simulink model "sm_bumper_car"  (R2021b)
settings: Solver=ode45  StartTime=0.0  StopTime=10.0  MaxStep=1e-3  RelTol=1e-3  AbsTol=1e-3
model workspace: external: MATLAB File sm_bumper_car_parameters.m (data not in the file)
values from neighbouring files (symbols this model uses):
  critical_velocity = 1e-2    (= 0.01)    [sm_bumper_car_parameters.m]
  damping = 30    [sm_bumper_car_parameters.m]
  g = 9.8    [sm_bumper_car_parameters.m]
  kinetic_friction_coef = 0.2    [sm_bumper_car_parameters.m]
  static_friction_coef = 0.2    [sm_bumper_car_parameters.m]
  stiffness = 10000    [sm_bumper_car_parameters.m]
  transition_region_width = 1e-5    (= 1e-05)    [sm_bumper_car_parameters.m]
undefined symbols (not defined in the file or in its folder): BackLeft, BackRight, BackStop, Body, car, EndRamp, FrontLeft, FrontRight, Incline, LeftRail, Ramp1, Ramp2, Ramp3, Ramp4, ramp_structure, RightRail, X, Y, Z
libraries: sm_lib x131, sm_bumper_car_lib x9, nesl_utility x1
(part 1 of 2)
Description:
  | Using the Spatial Contact Force Block - Bumper Car
settings Model: Creator=The MathWorks, Inc.  LastModifiedBy=The MathWorks, Inc.
settings SolverCC: AutoScaleAbsTol=off  AlgebraicLoopSolver=TrustRegion
settings DataIOCC: ReturnWorkspaceOutputs=off
settings DebuggingCC: SymbolicDimsDataTypeCodeGenerationDiagnostic=none  SFMachineParentedDataDiag=warning
settings SimscapeCC: SimscapeLogType=all  SimscapeLogSimulationStatistics=on  SimscapeLogName=simlog_sm_bumper_car  SimscapeLogDataHistory=20000
settings ExplorerConfigSet: InternalSimMechanicsExplorerSettings="<ExplorerConfiguration><canonicalview>default</canonicalview><AnimationSetting><BasePlaybackSpeed>1.0</BasePlaybackSpeed><PlaybackSpeedFactor>1.0</PlaybackSpeedFactor></AnimationSetting><TilePanel><TileInfo><Tiles Columns=\"1\" Count=\"1\" Rows=\"1\"><Column Weight=\"1\"/><Row Weight=\"1\"/><Tile Height=\"1\" Width=\"1\" X=\"0\" Y=\"0\"/></Tiles></TileInfo><SceneInfo><SceneViewer><BGColor><R>0.800000011920928955</R><G>0.800000011920928955</G><B>0.800000011920928955</B></BGColor><Camera><DoPerspective>off</DoPerspective><Position><X>0.637508295609907183</X><Y>-0.637508296451667844</Y><Z>1.11601012334107264</Z></Position><Center><X>-0.00639254054797280813</X><Y>0.00639253970621195267</Y><Z>0.472109287183192672</Z></Center><Up><X>-0.408248290463863073</X><Y>0.408248290463863073</Y><Z>0.816496580927726145</Z></Up><ViewLimDist>1</ViewLimDist><YLim>0.759088869094848628</YLim><XLim>0.995304530142192112</XLim></Camera></SceneViewer></SceneInfo></TilePanel><MechEditorPanel><Cameras/><GfxPanelCameraMap/><VideoCreator><PlaybackSpeedRatio>1.0</PlaybackSpeedRatio><FrameRate>30</FrameRate><VideoFormat>Motion JPEG AVI</VideoFormat><FrameSize>auto</FrameSize></VideoCreator></MechEditorPanel></ExplorerConfiguration>"

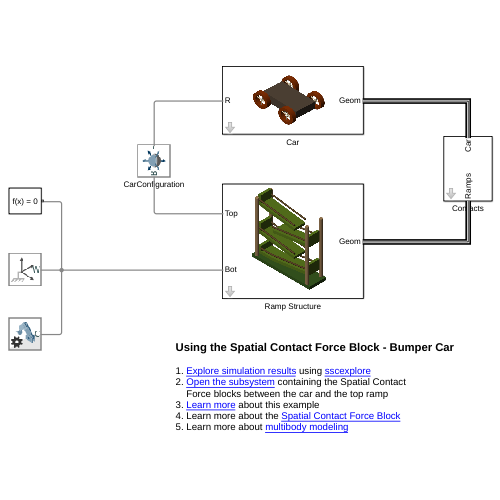
[thumbnail: Simulink's stored preview of the top-level diagram]
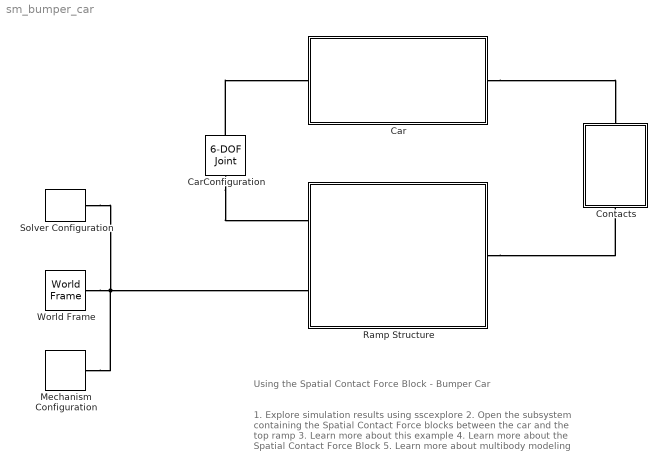
== system sm_bumper_car ==
  note: Using the Spatial Contact Force Block - Bumper Car
  note: 1. Explore simulation results using sscexplore
      | 2. Open the subsystem containing the Spatial Contact
      | Force blocks between the car and the top ramp
      | 3. Learn more about this example
      | 4. Learn more about the Spatial Contact Force Block
      | 5. Learn more about multibody modeling
  Car : Subsystem  mask{l=car.body.length, w=car.body.width, h=car.body.height, m=car.body.mass, body_color=car.body.color, wheel_radius=car.wheel.radius, wheel_width=car.wheel.thickness, wheel_m=car.wheel.mass, wheel_color=car.wheel.color, wheel_spoke_color=car.wheel.spoke.color}
      mask prompts: l "Length (cm)"; w "Width (cm)"; h "Height (cm)"; m "Body Mass (kg)"; body_color "Car Body Color"; wheel_radius "Radius"; wheel_width "Thickness"; wheel_m "Wheel Mass (kg)"; wheel_color "Wheel Color"; wheel_spoke_color "Wheel Spoke Color"
      mask init:
      | axle_len               = .85 * l;
      | axle_radius            = axle_len / 30;
      | wheel_inner_radius     = .67 * wheel_radius;
      | wheel_spoke_thickness = axle_radius / 2;
      | 
      | front_wheel_pos  = l * .12;
      | back_wheel_pos   = l * .88;
      | wheel_separation = axle_len;
      mask DialogControl BodyGroupVar Prompt: Body
      mask DialogControl BodyDimGroupVar Prompt: Dimensions
      mask DialogControl BodyInertiaGroupVar Prompt: Inertia
      mask DialogControl BodyGraphicGroupVar Prompt: Graphic
      mask DialogControl WheelGroupVar Prompt: Wheels
      mask DialogControl WheelDimGroupVar Prompt: Dimensions
      mask DialogControl WheelInertiaGroupVar Prompt: Inertia
      mask DialogControl WheelGraphicGroupVar Prompt: Graphic
      mask Display: image(fullfile(matlabroot,'toolbox','physmod','sm','smdemos','bumper_car','images','sm_bumper_car_car.png'));
  CarConfiguration : sm_lib/Joints/6-DOF Joint  JointMode=Normal  SenseConstraintForce=off  SenseConstraintForceX=off  SenseConstraintForceY=off  SenseConstraintForceZ=off  SenseConstraintTorque=off  SenseConstraintTorqueX=off  SenseConstraintTorqueY=off  SenseConstraintTorqueZ=off  SenseTotalForce=off  SenseTotalForceX=off  SenseTotalForceY=off  SenseTotalForceZ=off  SenseTotalTorque=off  SenseTotalTorqueX=off  SenseTotalTorqueY=off  SenseTotalTorqueZ=off  CompositeWrenchDir=FollowerOnBase  CompositeWrenchFrame=BaseFrame  PxEquilibriumPosition=0  PxEquilibriumPositionUnits=m  PxSpringStiffness=0  PxSpringStiffnessUnits=N/m  PxDampingCoefficient=0  PxDampingCoefficientUnits=N/(m/s)  PxTorqueActuationMode=NoTorque  PxMotionActuationMode=ComputedMotion  PxSensePosition=off  PxSenseVelocity=off  PxSenseAcceleration=off  PxSenseTorqueForce=off  PxSenseLowerLimitTorqueForce=off  PxSenseUpperLimitTorqueForce=off  PxLowerLimitSpecify=off  PxLowerLimitBound=-1  PxLowerLimitBoundUnits=m  PxLowerLimitStiffness=1e6  PxLowerLimitStiffnessUnits=N/m  PxLowerLimitDamping=1e3  PxLowerLimitDampingUnits=N/(m/s)  PxLowerLimitTransitionRegionWidth=1e-4  PxLowerLimitTransitionRegionWidthUnits=m  PxUpperLimitSpecify=off  PxUpperLimitBound=1  PxUpperLimitBoundUnits=m  PxUpperLimitStiffness=1e6  PxUpperLimitStiffnessUnits=N/m  PxUpperLimitDamping=1e3  PxUpperLimitDampingUnits=N/(m/s)  PxUpperLimitTransitionRegionWidth=1e-4  PxUpperLimitTransitionRegionWidthUnits=m  PxPositionTargetSpecify=on  PxPositionTargetPriority=High  PxPositionTargetValue=car.start_dist  PxPositionTargetValueUnits=cm  PxVelocityTargetSpecify=off  PxVelocityTargetPriority=High  PxVelocityTargetValue=0  PxVelocityTargetValueUnits=m/s  PyEquilibriumPosition=0  PyEquilibriumPositionUnits=m  PySpringStiffness=0  PySpringStiffnessUnits=N/m  PyDampingCoefficient=0  PyDampingCoefficientUnits=N/(m/s)  PyTorqueActuationMode=NoTorque  PyMotionActuationMode=ComputedMotion  PySensePosition=off  PySenseVelocity=off  PySenseAcceleration=off  PySenseTorqueForce=off  PySenseLowerLimitTorqueForce=off  PySenseUpperLimitTorqueForce=off  PyLowerLimitSpecify=off  PyLowerLimitBound=-1  PyLowerLimitBoundUnits=m  PyLowerLimitStiffness=1e6  PyLowerLimitStiffnessUnits=N/m  PyLowerLimitDamping=1e3  PyLowerLimitDampingUnits=N/(m/s)  PyLowerLimitTransitionRegionWidth=1e-4  PyLowerLimitTransitionRegionWidthUnits=m  PyUpperLimitSpecify=off  PyUpperLimitBound=1  PyUpperLimitBoundUnits=m  PyUpperLimitStiffness=1e6  PyUpperLimitStiffnessUnits=N/m  PyUpperLimitDamping=1e3  PyUpperLimitDampingUnits=N/(m/s)  PyUpperLimitTransitionRegionWidth=1e-4  PyUpperLimitTransitionRegionWidthUnits=m  PyPositionTargetSpecify=off  PyPositionTargetPriority=High  PyPositionTargetValue=0  PyPositionTargetValueUnits=m  PyVelocityTargetSpecify=off  PyVelocityTargetPriority=High  PyVelocityTargetValue=0  PyVelocityTargetValueUnits=m/s  PzEquilibriumPosition=0  PzEquilibriumPositionUnits=m  PzSpringStiffness=0  PzSpringStiffnessUnits=N/m  PzDampingCoefficient=0  PzDampingCoefficientUnits=N/(m/s)  PzTorqueActuationMode=NoTorque  PzMotionActuationMode=ComputedMotion  PzSensePosition=off  PzSenseVelocity=off  PzSenseAcceleration=off  PzSenseTorqueForce=off  PzSenseLowerLimitTorqueForce=off  PzSenseUpperLimitTorqueForce=off  PzLowerLimitSpecify=off  PzLowerLimitBound=-1  PzLowerLimitBoundUnits=m  PzLowerLimitStiffness=1e6  PzLowerLimitStiffnessUnits=N/m  PzLowerLimitDamping=1e3  PzLowerLimitDampingUnits=N/(m/s)  PzLowerLimitTransitionRegionWidth=1e-4  PzLowerLimitTransitionRegionWidthUnits=m  PzUpperLimitSpecify=off  PzUpperLimitBound=1  PzUpperLimitBoundUnits=m  PzUpperLimitStiffness=1e6  PzUpperLimitStiffnessUnits=N/m  PzUpperLimitDamping=1e3  PzUpperLimitDampingUnits=N/(m/s)  PzUpperLimitTransitionRegionWidth=1e-4  PzUpperLimitTransitionRegionWidthUnits=m  PzPositionTargetSpecify=on  PzPositionTargetPriority=High  PzPositionTargetValue=car.start_height  PzPositionTargetValueUnits=cm  PzVelocityTargetSpecify=off  PzVelocityTargetPriority=High  PzVelocityTargetValue=0  PzVelocityTargetValueUnits=m/s  SphDefPosRotationMethod=None  SphDefPosRotationAngleUnits=deg  SphDefPosRotationStandardAxis=+Z  SphDefPosRotationAngle=0.0  SphDefPosRotationArbitraryAxis=[0 0 1]  SphDefPosFollAlignAxisA=+X  SphDefPosBaseAlignAxisA=+Y  SphDefPosFollAlignAxisB=+Y  SphDefPosBaseAlignAxisB=+Z  SphDefPosRotationSequenceAxes=FollowerAxes  SphDefPosRotationSequence=XYX  SphDefPosRotationSequenceAngles=[0 0 0]  SphDefPosRotationSequenceAnglesUnits=deg  SphDefPosRotationMatrix=[1 0 0; 0 1 0; 0 0 1]  SphEqPosRotationMethod=None  SphEqPosRotationAngleUnits=deg  SphEqPosRotationStandardAxis=+Z  SphEqPosRotationAngle=0.0  SphEqPosRotationArbitraryAxis=[0 0 1]  SphEqPosFollAlignAxisA=+X  SphEqPosBaseAlignAxisA=+Y  SphEqPosFollAlignAxisB=+Y  SphEqPosBaseAlignAxisB=+Z  SphEqPosRotationSequenceAxes=FollowerAxes  SphEqPosRotationSequence=XYX  SphEqPosRotationSequenceAngles=[0 0 0]  SphEqPosRotationSequenceAnglesUnits=deg  SphEqPosRotationMatrix=[1 0 0; 0 1 0; 0 0 1]  SphSpringStiffness=0  SphSpringStiffnessUnits=N*m/deg  SphDampingCoefficient=0  SphDampingCoefficientUnits=N*m/(deg/s)  SphActuateTorqueX=off  SphActuateTorqueY=off  SphActuateTorqueZ=off  SphActuateTorque=off  SphTorqueActuationMode=NoTorque  SphMotionActuationMode=ComputedMotion  SphActuationFrame=BaseFrame  SphSensePosition=off  SphSenseVelocityX=off  SphSenseVelocityY=off  SphSenseVelocityZ=off  SphSenseVelocity=off  SphSenseAccelerationX=off  SphSenseAccelerationY=off  SphSenseAccelerationZ=off  SphSenseAcceleration=off  SphSenseTorqueX=off  SphSenseTorqueY=off  SphSenseTorqueZ=off  SphSenseTorqueForce=off  SphSenseLowerLimitTorqueMag=off  SphSenseUpperLimitTorqueMag=off  SphSensingFrame=BaseFrame  SphLowerLimitSpecify=off  SphLowerLimitBound=15  SphLowerLimitBoundUnits=deg  SphLowerLimitStiffness=1e4  SphLowerLimitStiffnessUnits=N*m/deg  SphLowerLimitDamping=10  SphLowerLimitDampingUnits=N*m/(deg/s)  SphLowerLimitTransitionRegionWidth=0.1  SphLowerLimitTransitionRegionWidthUnits=deg  SphUpperLimitSpecify=off  SphUpperLimitBound=45  SphUpperLimitBoundUnits=deg  SphUpperLimitStiffness=1e4  SphUpperLimitStiffnessUnits=N*m/deg  SphUpperLimitDamping=10  SphUpperLimitDampingUnits=N*m/(deg/s)  SphUpperLimitTransitionRegionWidth=0.1  SphUpperLimitTransitionRegionWidthUnits=deg  SphPositionTargetRotationMethod=StandardAxis  SphPositionTargetRotationAngleUnits=deg  SphPositionTargetRotationStandardAxis=-Y  SphPositionTargetRotationAngle=car.start_pitch  SphPositionTargetRotationArbitraryAxis=[0 0 1]  SphPositionTargetFollAlignAxisA=+X  SphPositionTargetBaseAlignAxisA=+Y  SphPositionTargetFollAlignAxisB=+Y  SphPositionTargetBaseAlignAxisB=+Z  SphPositionTargetRotationSequenceAxes=FollowerAxes  SphPositionTargetRotationSequence=XYX  SphPositionTargetRotationSequenceAngles=[0 0 0]  SphPositionTargetRotationSequenceAnglesUnits=deg  SphPositionTargetRotationMatrix=[1 0 0; 0 1 0; 0 0 1]  SphPositionTargetSpecify=on  SphPositionTargetPriority=High  SphVelocityTargetValue=[0 0 0]  SphVelocityTargetValueUnits=deg/s  SphVelocityTargetSpecify=off  SphVelocityTargetPriority=High  SphVelocityTargetInFollowerFrame=on
  Contacts : Subsystem  mask{k=stiffness, b=damping, tau=transition_region_width, mus=static_friction_coef, muk=kinetic_friction_coef, cv=critical_velocity}
      mask prompts: k "Stiffness (N/m)"; b "Damping (N/(m/s))"; tau "Transition Region Width (m)"; mus "Coefficient of Static Friction"; muk "Coefficient of Kinetic Friction"; cv "Critical Velocity (m/s)"
  Mechanism Configuration : sm_lib/Utilities/Mechanism Configuration  UniformGravity=Constant  GravityVector=[0 0 -g]  GravityUnits=m/s^2  LinearizationDelta=0.001  JointModeTransitionNonlinearIterations=2
  Ramp Structure : Subsystem  mask{w=ramp_structure.width, l=ramp_structure.length, ramp_angle=ramp_structure.ramp.angle, surface_color=ramp_structure.ramp.color, rail_color=ramp_structure.rail.color, pillar_color=ramp_structure.pillar.color, base_color=ramp_structure.base.color}
      mask prompts: w "Width (cm)"; l "Length (cm)"; ramp_angle "Ramp Angle (deg)"; surface_color "Surface Color"; rail_color "Rail Color"; pillar_color "Pillar Color"; base_color "Base Color"
      mask init:
      | ramp.angle = ramp_angle;
      | theta_ = deg2rad(ramp.angle);
      | 
      | ramp.w       = w;
      | ramp.h       = ramp.w / 4;
      | 
      | wall.h        = ramp.w;
      | 
      | dropoff_h     = .75 * ramp.w;
      | dropoff_dist  = 1.5 * ramp.w;
      | 
      | ramp.l        = (l - dropoff_dist - sin(theta_)*ramp.h/2)...
      |                 / cos(theta_);
      | 
      | rail.r        = .28 * ramp.h;
      | rail.l        = ramp.l;
      | 
      | rail.h = 1.5 * ramp.h;
      | 
      | end_ramp.l = dropoff_dist + ramp.h;
      | 
      | ramp.w = ramp.w + 2 * rail.r;
      mask DialogControl ParameterGroupVar Prompt: Geometry
      mask DialogControl GraphicsGroupVar Prompt: Graphic
      mask Display: image(fullfile(matlabroot,'toolbox','physmod','sm','smdemos','bumper_car','images','sm_bumper_car_ramp_structure.png'));
  Solver Configuration : nesl_utility/Solver Configuration  PhysicalDomain=network_engine_domain  SubClassName=solver  LeftPortType=input  RightPortType=generic  Tones=[]  Harmonics=[]  SimulateNoise=off  Profile=off  UseLocalSampling=off  EnableSwitchedLinearOptims=on  FrequencyDomain=off  UseCCode=off  RelTol=0.001  AbsTol=1e-06  MinStep=1e-09  ToWorkspace=off  RevertToSquareIcSolve=off  NumHomotopyIterations=100  PhasorMode=off  PhasorModeNumHarmonics=1  DoDC=off  ResidualTolerance=1e-09  UseLocalSolver=off  LocalSolverChoice=NE_BACKWARD_EULER_ADVANCER  LocalSolverSampleTime=0.001  DoFixedCost=off  MaxNonlinIter=3  MaxModeIter=2  ComputeImpulses=off  ImpulseIterations=2  LinearAlgebra=Sparse  EquationFormulation=NE_TIME_EF  DelaysMemoryBudget=1024  AutomaticFiltering=on  FilteringTimeConstant=0.001  PartitionStorageMethod=AS_NEEDED  PartitionMemoryBudget=1024  PartitionMethod=FAST
      settings: SourceProductBaseCode=PW,SS
  World Frame : sm_lib/Frames and Transforms/World Frame
  connections:
  Solver Configuration/RConn1 -- Ramp Structure/LConn2 -- Mechanism Configuration/RConn1 -- World Frame/RConn1
  CarConfiguration/RConn1 -- Car/LConn1
  CarConfiguration/LConn1 -- Ramp Structure/LConn1
  Ramp Structure/RConn1 -- Contacts/LConn1
  Car/RConn1 -- Contacts/RConn1

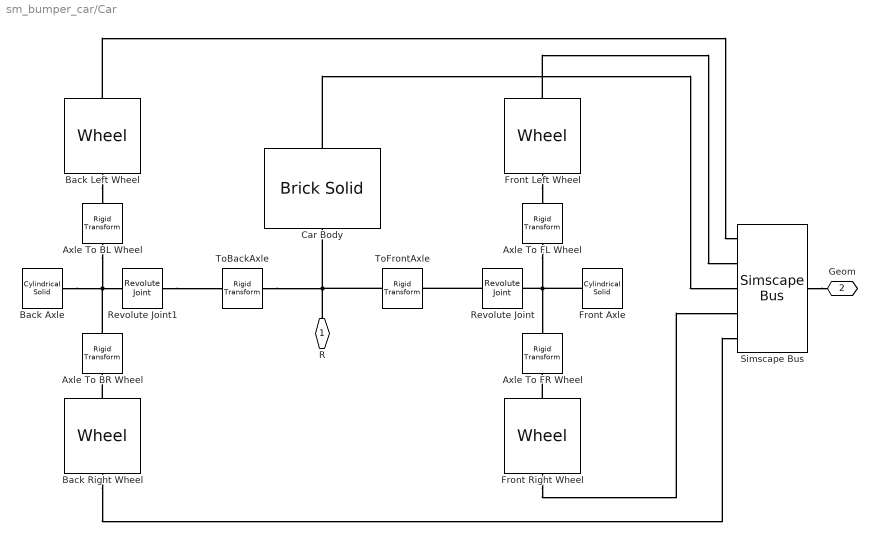
== system sm_bumper_car/Car ==
  Axle To BL Wheel : sm_lib/Frames and Transforms/Rigid Transform  TranslationMethod=StandardAxis  TranslationStandardOffset=wheel_separation/2  TranslationLengthUnit=cm  TranslationStandardAxis=-Z  TranslationCartesianOffset=[0 0 0]  TranslationROffset=0  TranslationROffsetUnits=m  TranslationZOffset=0  TranslationZOffsetUnits=m  TranslationThetaOffset=0  TranslationThetaOffsetUnits=deg  RotationMethod=None  RotationAngleUnits=deg  RotationStandardAxis=+Z  RotationAngle=0.0  RotationArbitraryAxis=[0 0 1]  FollAlignAxisA=+X  BaseAlignAxisA=+Y  FollAlignAxisB=+Y  BaseAlignAxisB=+Z  RotationSequenceAxes=FollowerAxes  RotationSequence=XYX  RotationSequenceAngles=[0 0 0]  RotationSequenceAnglesUnits=deg  RotationMatrix=[1 0 0; 0 1 0; 0 0 1]
  Axle To BR Wheel : sm_lib/Frames and Transforms/Rigid Transform  TranslationMethod=StandardAxis  TranslationStandardOffset=wheel_separation/2  TranslationLengthUnit=cm  TranslationStandardAxis=+Z  TranslationCartesianOffset=[0 0 0]  TranslationROffset=0  TranslationROffsetUnits=m  TranslationZOffset=0  TranslationZOffsetUnits=m  TranslationThetaOffset=0  TranslationThetaOffsetUnits=deg  RotationMethod=None  RotationAngleUnits=deg  RotationStandardAxis=+Z  RotationAngle=0.0  RotationArbitraryAxis=[0 0 1]  FollAlignAxisA=+X  BaseAlignAxisA=+Y  FollAlignAxisB=+Y  BaseAlignAxisB=+Z  RotationSequenceAxes=FollowerAxes  RotationSequence=XYX  RotationSequenceAngles=[0 0 0]  RotationSequenceAnglesUnits=deg  RotationMatrix=[1 0 0; 0 1 0; 0 0 1]
  Axle To FL Wheel : sm_lib/Frames and Transforms/Rigid Transform  TranslationMethod=StandardAxis  TranslationStandardOffset=wheel_separation/2  TranslationLengthUnit=cm  TranslationStandardAxis=-Z  TranslationCartesianOffset=[0 0 0]  TranslationROffset=0  TranslationROffsetUnits=m  TranslationZOffset=0  TranslationZOffsetUnits=m  TranslationThetaOffset=0  TranslationThetaOffsetUnits=deg  RotationMethod=None  RotationAngleUnits=deg  RotationStandardAxis=+Z  RotationAngle=0.0  RotationArbitraryAxis=[0 0 1]  FollAlignAxisA=+X  BaseAlignAxisA=+Y  FollAlignAxisB=+Y  BaseAlignAxisB=+Z  RotationSequenceAxes=FollowerAxes  RotationSequence=XYX  RotationSequenceAngles=[0 0 0]  RotationSequenceAnglesUnits=deg  RotationMatrix=[1 0 0; 0 1 0; 0 0 1]
  Axle To FR Wheel : sm_lib/Frames and Transforms/Rigid Transform  TranslationMethod=StandardAxis  TranslationStandardOffset=wheel_separation/2  TranslationLengthUnit=cm  TranslationStandardAxis=+Z  TranslationCartesianOffset=[0 0 0]  TranslationROffset=0  TranslationROffsetUnits=m  TranslationZOffset=0  TranslationZOffsetUnits=m  TranslationThetaOffset=0  TranslationThetaOffsetUnits=deg  RotationMethod=None  RotationAngleUnits=deg  RotationStandardAxis=+Z  RotationAngle=0.0  RotationArbitraryAxis=[0 0 1]  FollAlignAxisA=+X  BaseAlignAxisA=+Y  FollAlignAxisB=+Y  BaseAlignAxisB=+Z  RotationSequenceAxes=FollowerAxes  RotationSequence=XYX  RotationSequenceAngles=[0 0 0]  RotationSequenceAnglesUnits=deg  RotationMatrix=[1 0 0; 0 1 0; 0 0 1]
  Back Axle : sm_lib/Body Elements/Cylindrical Solid  GraphicAmbientColor=[0.15 0.15 0.15 1.0]  BasedOnType=Density  CenterOfMass=[0 0 0]  CenterOfMassUnits=m  GraphicDiffuseColor=wheel_spoke_color  CylinderLength=axle_len  CylinderLengthUnits=cm  CylinderRadius=axle_radius  CylinderRadiusUnits=cm  Density=0  DensityUnits=kg/m^3  DoExposeReferenceFrame=on  GraphicEmissiveColor=[0.0 0.0 0.0 1.0]  ExportEntireGeometry=off  SerializedFrames=<Frames/>  MarkerShape=Sphere  MarkerSize=10  GraphicType=FromGeometry  InertiaType=CalculateFromGeometry  Mass=1  MassUnits=kg  MomentsOfInertia=[1 1 1]  MomentsOfInertiaUnits=kg*m^2  GraphicOpacity=1.0  ProductsOfInertia=[0 0 0]  ProductsOfInertiaUnits=kg*m^2  GraphicShininess=75  GraphicSpecularColor=[0.5 0.5 0.5 1.0]  GraphicVisPropType=SimpleVisualProperties
  Back Left Wheel : sm_bumper_car_lib/Wheel  r=wheel_radius  rin=wheel_inner_radius  spoke_r=wheel_spoke_thickness  W=wheel_width  m=wheel_m  color=wheel_color  spoke_color=wheel_spoke_color
      settings: SourceProductBaseCode=MS
  Back Right Wheel : sm_bumper_car_lib/Wheel  r=wheel_radius  rin=wheel_inner_radius  spoke_r=wheel_spoke_thickness  W=wheel_width  m=wheel_m  color=wheel_color  spoke_color=wheel_spoke_color
      settings: SourceProductBaseCode=MS
  Car Body : sm_lib/Body Elements/Brick Solid  GraphicAmbientColor=[0.15 0.15 0.15 1.0]  BasedOnType=Mass  BrickDimensions=[l w h]  BrickDimensionUnits=cm  CenterOfMass=[0 0 0]  CenterOfMassUnits=cm  GraphicDiffuseColor=body_color  Density=1000  DensityUnits=kg/m^3  DoExposeReferenceFrame=on  GraphicEmissiveColor=[0.0 0.0 0.0 1.0]  ExportEntireGeometry=on  SerializedFrames=<Frames/>  MarkerShape=Sphere  MarkerSize=10  GraphicType=FromGeometry  InertiaType=CalculateFromGeometry  Mass=m  MassUnits=kg  MomentsOfInertia=[1 1 1]  MomentsOfInertiaUnits=kg*m^2  GraphicOpacity=1.0  ProductsOfInertia=[0 0 0]  ProductsOfInertiaUnits=kg*m^2  GraphicShininess=75  GraphicSpecularColor=[0.5 0.5 0.5 1.0]  GraphicVisPropType=SimpleVisualProperties
  Front Axle : sm_lib/Body Elements/Cylindrical Solid  GraphicAmbientColor=[0.15 0.15 0.15 1.0]  BasedOnType=Density  CenterOfMass=[0 0 0]  CenterOfMassUnits=m  GraphicDiffuseColor=wheel_spoke_color  CylinderLength=axle_len  CylinderLengthUnits=cm  CylinderRadius=axle_radius  CylinderRadiusUnits=cm  Density=0  DensityUnits=kg/m^3  DoExposeReferenceFrame=on  GraphicEmissiveColor=[0.0 0.0 0.0 1.0]  ExportEntireGeometry=off  SerializedFrames=<Frames/>  MarkerShape=Sphere  MarkerSize=10  GraphicType=FromGeometry  InertiaType=CalculateFromGeometry  Mass=1  MassUnits=kg  MomentsOfInertia=[1 1 1]  MomentsOfInertiaUnits=kg*m^2  GraphicOpacity=1.0  ProductsOfInertia=[0 0 0]  ProductsOfInertiaUnits=kg*m^2  GraphicShininess=75  GraphicSpecularColor=[0.5 0.5 0.5 1.0]  GraphicVisPropType=SimpleVisualProperties
  Front Left Wheel : sm_bumper_car_lib/Wheel  r=wheel_radius  rin=wheel_inner_radius  spoke_r=wheel_spoke_thickness  W=wheel_width  m=wheel_m  color=wheel_color  spoke_color=wheel_spoke_color
      settings: SourceProductBaseCode=MS
  Front Right Wheel : sm_bumper_car_lib/Wheel  r=wheel_radius  rin=wheel_inner_radius  spoke_r=wheel_spoke_thickness  W=wheel_width  m=wheel_m  color=wheel_color  spoke_color=wheel_spoke_color
      settings: SourceProductBaseCode=MS
  Revolute Joint : sm_lib/Joints/Revolute Joint  JointMode=Normal  SenseConstraintForce=off  SenseConstraintForceX=off  SenseConstraintForceY=off  SenseConstraintForceZ=off  SenseConstraintTorque=off  SenseConstraintTorqueX=off  SenseConstraintTorqueY=off  SenseConstraintTorqueZ=off  SenseTotalForce=off  SenseTotalForceX=off  SenseTotalForceY=off  SenseTotalForceZ=off  SenseTotalTorque=off  SenseTotalTorqueX=off  SenseTotalTorqueY=off  SenseTotalTorqueZ=off  CompositeWrenchDir=FollowerOnBase  CompositeWrenchFrame=BaseFrame  EquilibriumPosition=0  EquilibriumPositionUnits=deg  SpringStiffness=0  SpringStiffnessUnits=N*m/deg  DampingCoefficient=0  DampingCoefficientUnits=N*m/(deg/s)  TorqueActuationMode=NoTorque  MotionActuationMode=ComputedMotion  SensePosition=off  SenseVelocity=off  SenseAcceleration=off  SenseTorqueForce=off  SenseLowerLimitTorqueForce=off  SenseUpperLimitTorqueForce=off  LowerLimitSpecify=off  LowerLimitBound=-90  LowerLimitBoundUnits=deg  LowerLimitStiffness=1e4  LowerLimitStiffnessUnits=N*m/deg  LowerLimitDamping=10  LowerLimitDampingUnits=N*m/(deg/s)  LowerLimitTransitionRegionWidth=0.1  LowerLimitTransitionRegionWidthUnits=deg  UpperLimitSpecify=off  UpperLimitBound=90  UpperLimitBoundUnits=deg  UpperLimitStiffness=1e4  UpperLimitStiffnessUnits=N*m/deg  UpperLimitDamping=10  UpperLimitDampingUnits=N*m/(deg/s)  UpperLimitTransitionRegionWidth=0.1  UpperLimitTransitionRegionWidthUnits=deg  PositionTargetSpecify=off  PositionTargetPriority=High  PositionTargetValue=0  PositionTargetValueUnits=deg  VelocityTargetSpecify=off  VelocityTargetPriority=High  VelocityTargetValue=0  VelocityTargetValueUnits=deg/s
  Revolute Joint1 : sm_lib/Joints/Revolute Joint  JointMode=Normal  SenseConstraintForce=off  SenseConstraintForceX=off  SenseConstraintForceY=off  SenseConstraintForceZ=off  SenseConstraintTorque=off  SenseConstraintTorqueX=off  SenseConstraintTorqueY=off  SenseConstraintTorqueZ=off  SenseTotalForce=off  SenseTotalForceX=off  SenseTotalForceY=off  SenseTotalForceZ=off  SenseTotalTorque=off  SenseTotalTorqueX=off  SenseTotalTorqueY=off  SenseTotalTorqueZ=off  CompositeWrenchDir=FollowerOnBase  CompositeWrenchFrame=BaseFrame  EquilibriumPosition=0  EquilibriumPositionUnits=deg  SpringStiffness=0  SpringStiffnessUnits=N*m/deg  DampingCoefficient=0  DampingCoefficientUnits=N*m/(deg/s)  TorqueActuationMode=NoTorque  MotionActuationMode=ComputedMotion  SensePosition=off  SenseVelocity=off  SenseAcceleration=off  SenseTorqueForce=off  SenseLowerLimitTorqueForce=off  SenseUpperLimitTorqueForce=off  LowerLimitSpecify=off  LowerLimitBound=-90  LowerLimitBoundUnits=deg  LowerLimitStiffness=1e4  LowerLimitStiffnessUnits=N*m/deg  LowerLimitDamping=10  LowerLimitDampingUnits=N*m/(deg/s)  LowerLimitTransitionRegionWidth=0.1  LowerLimitTransitionRegionWidthUnits=deg  UpperLimitSpecify=off  UpperLimitBound=90  UpperLimitBoundUnits=deg  UpperLimitStiffness=1e4  UpperLimitStiffnessUnits=N*m/deg  UpperLimitDamping=10  UpperLimitDampingUnits=N*m/(deg/s)  UpperLimitTransitionRegionWidth=0.1  UpperLimitTransitionRegionWidthUnits=deg  PositionTargetSpecify=off  PositionTargetPriority=High  PositionTargetValue=0  PositionTargetValueUnits=deg  VelocityTargetSpecify=off  VelocityTargetPriority=High  VelocityTargetValue=0  VelocityTargetValueUnits=deg/s
  Simscape Bus : SimscapeBus  HierarchyStrings=BackLeft;FrontLeft;Body;FrontRight;BackRight
  ToBackAxle : sm_lib/Frames and Transforms/Rigid Transform  TranslationMethod=StandardAxis  TranslationStandardOffset=l/2 - back_wheel_pos  TranslationLengthUnit=cm  TranslationStandardAxis=+X  TranslationCartesianOffset=[0 0 0]  TranslationROffset=0  TranslationROffsetUnits=m  TranslationZOffset=0  TranslationZOffsetUnits=m  TranslationThetaOffset=0  TranslationThetaOffsetUnits=deg  RotationMethod=AlignedAxes  RotationAngleUnits=deg  RotationStandardAxis=+Z  RotationAngle=0.0  RotationArbitraryAxis=[0 0 1]  FollAlignAxisA=+Y  BaseAlignAxisA=+Z  FollAlignAxisB=+Z  BaseAlignAxisB=-Y  RotationSequenceAxes=FollowerAxes  RotationSequence=XYX  RotationSequenceAngles=[0 0 0]  RotationSequenceAnglesUnits=deg  RotationMatrix=[1 0 0; 0 1 0; 0 0 1]
  ToFrontAxle : sm_lib/Frames and Transforms/Rigid Transform  TranslationMethod=StandardAxis  TranslationStandardOffset=l/2 - front_wheel_pos  TranslationLengthUnit=cm  TranslationStandardAxis=+X  TranslationCartesianOffset=[0 0 0]  TranslationROffset=0  TranslationROffsetUnits=m  TranslationZOffset=0  TranslationZOffsetUnits=m  TranslationThetaOffset=0  TranslationThetaOffsetUnits=deg  RotationMethod=AlignedAxes  RotationAngleUnits=deg  RotationStandardAxis=+Z  RotationAngle=0.0  RotationArbitraryAxis=[0 0 1]  FollAlignAxisA=+Y  BaseAlignAxisA=+Z  FollAlignAxisB=+Z  BaseAlignAxisB=-Y  RotationSequenceAxes=FollowerAxes  RotationSequence=XYX  RotationSequenceAngles=[0 0 0]  RotationSequenceAnglesUnits=deg  RotationMatrix=[1 0 0; 0 1 0; 0 0 1]
  R : PMIOPort  Side=Left
  Geom : PMIOPort  Port=2  Side=Right
  connections:
  Back Right Wheel/LConn1 -- Axle To BR Wheel/RConn1
  ToFrontAxle/LConn1 -- Car Body/RConn1 -- R/RConn1 -- ToBackAxle/LConn1
  Front Left Wheel/LConn1 -- Axle To FL Wheel/RConn1
  Revolute Joint1/LConn1 -- ToBackAxle/RConn1
  Revolute Joint/LConn1 -- ToFrontAxle/RConn1
  Axle To FL Wheel/LConn1 -- Front Axle/RConn1 -- Axle To FR Wheel/LConn1 -- Revolute Joint/RConn1
  Axle To BR Wheel/LConn1 -- Back Axle/RConn1 -- Axle To BL Wheel/LConn1 -- Revolute Joint1/RConn1
  Front Right Wheel/LConn1 -- Axle To FR Wheel/RConn1
  Back Left Wheel/LConn1 -- Axle To BL Wheel/RConn1
  Simscape Bus/RConn1 -- Geom/RConn1
  Car Body/LConn1 -- Simscape Bus/LConn3
  Front Left Wheel/RConn1 -- Simscape Bus/LConn2
  Back Left Wheel/RConn1 -- Simscape Bus/LConn1
  Front Right Wheel/RConn1 -- Simscape Bus/LConn4
  Back Right Wheel/RConn1 -- Simscape Bus/LConn5

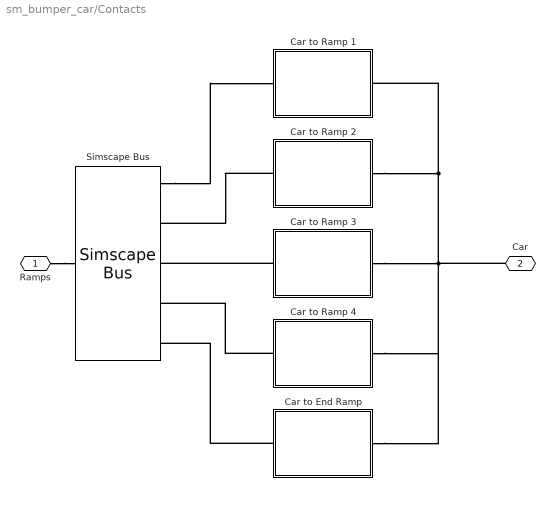
== system sm_bumper_car/Contacts ==
  Car to End Ramp : Subsystem
  Car to Ramp 1 : Subsystem
  Car to Ramp 2 : Subsystem
  Car to Ramp 3 : Subsystem
  Car to Ramp 4 : Subsystem
  Simscape Bus : SimscapeBus  HierarchyStrings=Ramp1;Ramp2;Ramp3;Ramp4;EndRamp
  Ramps : PMIOPort  Side=Left
  Car : PMIOPort  Port=2  Side=Right
  connections:
  Ramps/RConn1 -- Simscape Bus/RConn1
  Simscape Bus/LConn1 -- Car to Ramp 1/LConn1
  Car to Ramp 2/LConn1 -- Simscape Bus/LConn2
  Car to Ramp 3/LConn1 -- Simscape Bus/LConn3
  Car to Ramp 4/LConn1 -- Simscape Bus/LConn4
  Car to End Ramp/LConn1 -- Simscape Bus/LConn5
  Car/RConn1 -- Car to Ramp 3/RConn1 -- Car to End Ramp/RConn1 -- Car to Ramp 4/RConn1 -- Car to Ramp 2/RConn1 -- Car to Ramp 1/RConn1

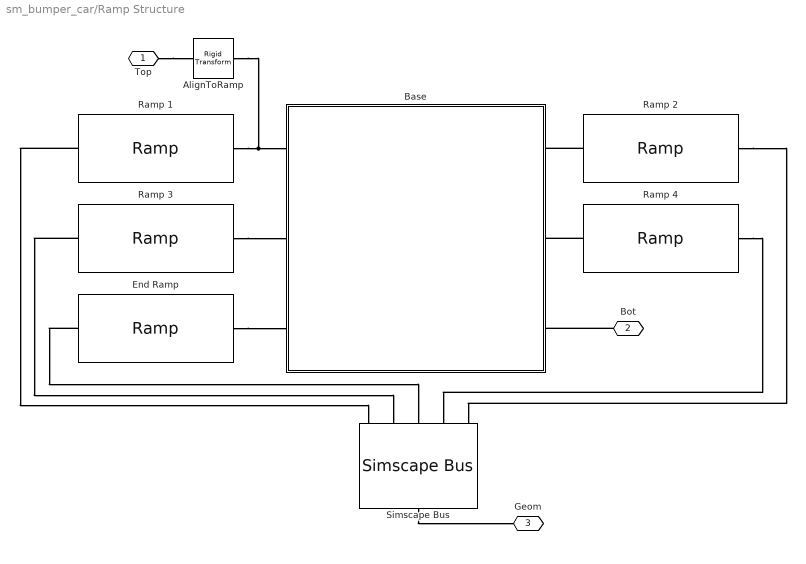
== system sm_bumper_car/Ramp Structure ==
  AlignToRamp : sm_lib/Frames and Transforms/Rigid Transform  TranslationMethod=None  TranslationStandardOffset=0  TranslationLengthUnit=cm  TranslationStandardAxis=+Z  TranslationCartesianOffset=[0 0 0]  TranslationROffset=0  TranslationROffsetUnits=m  TranslationZOffset=0  TranslationZOffsetUnits=m  TranslationThetaOffset=0  TranslationThetaOffsetUnits=deg  RotationMethod=StandardAxis  RotationAngleUnits=deg  RotationStandardAxis=+Y  RotationAngle=ramp_angle  RotationArbitraryAxis=[0 0 1]  FollAlignAxisA=+X  BaseAlignAxisA=+Y  FollAlignAxisB=+Y  BaseAlignAxisB=+Z  RotationSequenceAxes=FollowerAxes  RotationSequence=XYX  RotationSequenceAngles=[0 0 0]  RotationSequenceAnglesUnits=deg  RotationMatrix=[1 0 0; 0 1 0; 0 0 1]
  Base : Subsystem  mask{width=w, length=l, ramp_length=ramp.l, ramp_width=ramp.w, ramp_height=ramp.h, backstop_height=wall.h, ramp_angle=ramp.angle, rail_radius=rail.r, dropoff_height=dropoff_h}
      mask prompts: width "Width (cm)"; length "Length (cm)"; ramp_length "Ramp Length (cm)"; ramp_width "Ramp Width (cm)"; ramp_height "Ramp Height (cm)"; backstop_height "Back Stop Height (cm)"; ramp_angle "Ramp Angle (degrees)"; rail_radius "Rail Radius (cm)"; dropoff_height "Dropoff Height (cm)"
      mask init:
      | theta_ = deg2rad(ramp_angle);
      | 
      | ramp_vert_height    = ramp_length * sin(theta_);
      | 
      | pillar_height       = 4 * ramp_vert_height...
      |                       + 3 * dropoff_height...
      |                       + 4 * ramp_height;
      | 
      | pillar_width        = 2.2 * rail_radius;
      | contraption_length  = length;      % distance between opposite support
      |                                    % pillars
      | base_length         = contraption_length + 15;
      | base_width          = ramp_width + 4 * pillar_width;
      | base_height         = .28 * width;
      mask Display: image(fullfile(matlabroot,'toolbox','physmod','sm','smdemos','bumper_car','images','sm_bumper_car_support_pillars.png'));
  End Ramp : sm_bumper_car_lib/Ramp  L=end_ramp.l  W=ramp.w  H=ramp.h  wall_h=wall.h  incline=0  rail_r=rail.r  rail_l=end_ramp.l  rail_h=rail.h  color=surface_color  rail_color=rail_color
      settings: SourceProductBaseCode=MS
  Ramp {1..4} (4 alike) : sm_bumper_car_lib/Ramp  L=ramp.l  W=ramp.w  H=ramp.h  wall_h=wall.h  incline=ramp.angle  rail_r=rail.r  rail_l=rail.l  rail_h=rail.h  color=surface_color  rail_color=rail_color
      settings: SourceProductBaseCode=MS
  Simscape Bus : SimscapeBus  HierarchyStrings=Ramp1;Ramp3;EndRamp;Ramp4;Ramp2
  Top : PMIOPort  Side=Left
  Bot : PMIOPort  Port=2  Side=Left
  Geom : PMIOPort  Port=3  Side=Right
  connections:
  Simscape Bus/RConn1 -- Geom/RConn1
  Top/RConn1 -- AlignToRamp/RConn1
  Bot/RConn1 -- Base/RConn3
  Ramp 4/LConn1 -- Base/RConn2
  Ramp 2/LConn1 -- Base/RConn1
  End Ramp/LConn1 -- Base/LConn3
  Ramp 3/LConn1 -- Base/LConn2
  Ramp 1/LConn1 -- AlignToRamp/LConn1 -- Base/LConn1
  Ramp 4/RConn1 -- Simscape Bus/LConn4
  Ramp 1/RConn1 -- Simscape Bus/LConn1
  Ramp 3/RConn1 -- Simscape Bus/LConn2
  End Ramp/RConn1 -- Simscape Bus/LConn3
  Ramp 2/RConn1 -- Simscape Bus/LConn5

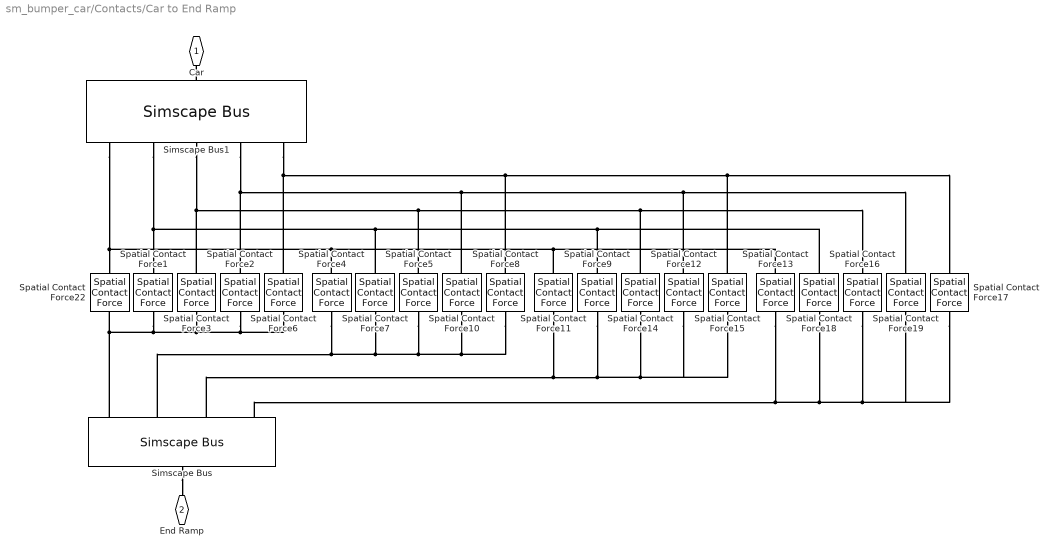
== system sm_bumper_car/Contacts/Car to End Ramp ==
  Simscape Bus : SimscapeBus  HierarchyStrings=Incline;BackStop;LeftRail;RightRail
  Simscape Bus1 : SimscapeBus  HierarchyStrings=Body;BackLeft;BackRight;FrontLeft;FrontRight
  Spatial Contact Force{1..19,22} (20 alike) : sm_lib/Forces and Torques/Spatial Contact Force  CoefficientOfDynamicFriction=muk  CoefficientOfStaticFriction=mus  SenseContactBaseRotation=off  SenseContactBaseTranslation=off  NormalDamping=b  NormalDampingUnits=N/(m/s)  SenseContactFollowerRotation=off  SenseContactFollowerTranslation=off  SenseContactSignal=off  NormalStiffness=k  NormalStiffnessUnits=N/m  FrictionalCriticalVelocity=cv  FrictionalCriticalVelocityUnits=m/s  ZeroCrossDetectContactStartAndEnd=off  FrictionType=SmoothStickSlip  SenseFrictionalForceMagnitude=off  SenseNormalForceMagnitude=off  NormalForceType=SmoothSpringDamper  SenseNormalVelocity=off  SenseSeparationDistance=off  SenseTangentialVelocity=off  SenseTangentialVelocityMagnitude=off  NormalTransitionRegionWidth=tau  NormalTransitionRegionWidthUnits=m
  Car : PMIOPort  Side=Right
  End Ramp : PMIOPort  Port=2  Side=Left
  connections:
  Simscape Bus1/LConn5 -- Spatial Contact Force6/RConn1 -- Spatial Contact Force8/RConn1 -- Spatial Contact Force17/RConn1 -- Spatial Contact Force15/RConn1
  Spatial Contact Force2/RConn1 -- Simscape Bus1/LConn4 -- Spatial Contact Force10/RConn1 -- Spatial Contact Force19/RConn1 -- Spatial Contact Force12/RConn1
  Spatial Contact Force3/RConn1 -- Spatial Contact Force5/RConn1 -- Spatial Contact Force14/RConn1 -- Spatial Contact Force16/RConn1 -- Simscape Bus1/LConn3
  Spatial Contact Force18/RConn1 -- Spatial Contact Force9/RConn1 -- Spatial Contact Force7/RConn1 -- Simscape Bus1/LConn2 -- Spatial Contact Force1/RConn1
  Spatial Contact Force11/RConn1 -- Spatial Contact Force13/RConn1 -- Spatial Contact Force4/RConn1 -- Simscape Bus1/LConn1 -- Spatial Contact Force22/RConn1
  Simscape Bus1/RConn1 -- Car/RConn1
  Simscape Bus/RConn1 -- End Ramp/RConn1
  Spatial Contact Force18/LConn1 -- Spatial Contact Force17/LConn1 -- Spatial Contact Force19/LConn1 -- Spatial Contact Force16/LConn1 -- Spatial Contact Force13/LConn1 -- Simscape Bus/LConn4
  Spatial Contact Force11/LConn1 -- Simscape Bus/LConn3 -- Spatial Contact Force9/LConn1 -- Spatial Contact Force15/LConn1 -- Spatial Contact Force12/LConn1 -- Spatial Contact Force14/LConn1
  Spatial Contact Force10/LConn1 -- Spatial Contact Force8/LConn1 -- Spatial Contact Force5/LConn1 -- Spatial Contact Force7/LConn1 -- Spatial Contact Force4/LConn1 -- Simscape Bus/LConn2
  Spatial Contact Force2/LConn1 -- Spatial Contact Force6/LConn1 -- Simscape Bus/LConn1 -- Spatial Contact Force22/LConn1 -- Spatial Contact Force1/LConn1 -- Spatial Contact Force3/LConn1

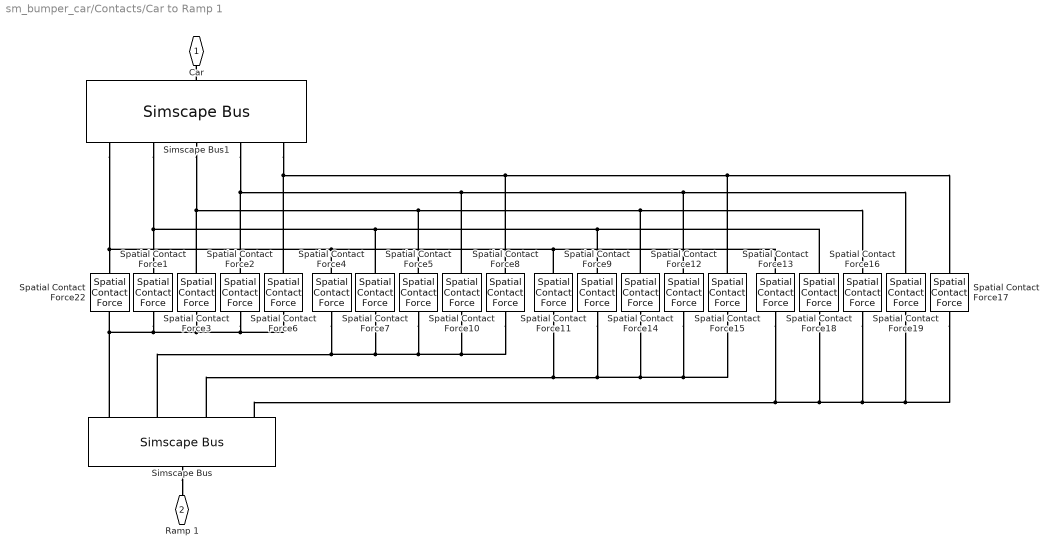
== system sm_bumper_car/Contacts/Car to Ramp 1 ==
  Simscape Bus : SimscapeBus  HierarchyStrings=Incline;BackStop;LeftRail;RightRail
  Simscape Bus1 : SimscapeBus  HierarchyStrings=Body;BackLeft;BackRight;FrontLeft;FrontRight
  Spatial Contact Force{1..19,22} (20 alike) : sm_lib/Forces and Torques/Spatial Contact Force  CoefficientOfDynamicFriction=muk  CoefficientOfStaticFriction=mus  SenseContactBaseRotation=off  SenseContactBaseTranslation=off  NormalDamping=b  NormalDampingUnits=N/(m/s)  SenseContactFollowerRotation=off  SenseContactFollowerTranslation=off  SenseContactSignal=off  NormalStiffness=k  NormalStiffnessUnits=N/m  FrictionalCriticalVelocity=cv  FrictionalCriticalVelocityUnits=m/s  ZeroCrossDetectContactStartAndEnd=off  FrictionType=SmoothStickSlip  SenseFrictionalForceMagnitude=off  SenseNormalForceMagnitude=off  NormalForceType=SmoothSpringDamper  SenseNormalVelocity=off  SenseSeparationDistance=off  SenseTangentialVelocity=off  SenseTangentialVelocityMagnitude=off  NormalTransitionRegionWidth=tau  NormalTransitionRegionWidthUnits=m
  Car : PMIOPort  Side=Right
  Ramp 1 : PMIOPort  Port=2  Side=Left
  connections:
  Spatial Contact Force22/LConn1 -- Simscape Bus/LConn1 -- Spatial Contact Force6/LConn1 -- Spatial Contact Force2/LConn1 -- Spatial Contact Force3/LConn1 -- Spatial Contact Force1/LConn1
  Simscape Bus/LConn2 -- Spatial Contact Force10/LConn1 -- Spatial Contact Force8/LConn1 -- Spatial Contact Force5/LConn1 -- Spatial Contact Force7/LConn1 -- Spatial Contact Force4/LConn1
  Simscape Bus/LConn3 -- Spatial Contact Force11/LConn1 -- Spatial Contact Force14/LConn1 -- Spatial Contact Force12/LConn1 -- Spatial Contact Force15/LConn1 -- Spatial Contact Force9/LConn1
  Simscape Bus/LConn4 -- Spatial Contact Force18/LConn1 -- Spatial Contact Force16/LConn1 -- Spatial Contact Force19/LConn1 -- Spatial Contact Force17/LConn1 -- Spatial Contact Force13/LConn1
  Simscape Bus/RConn1 -- Ramp 1/RConn1
  Simscape Bus1/RConn1 -- Car/RConn1
  Simscape Bus1/LConn1 -- Spatial Contact Force13/RConn1 -- Spatial Contact Force11/RConn1 -- Spatial Contact Force4/RConn1 -- Spatial Contact Force22/RConn1
  Simscape Bus1/LConn2 -- Spatial Contact Force9/RConn1 -- Spatial Contact Force18/RConn1 -- Spatial Contact Force7/RConn1 -- Spatial Contact Force1/RConn1
  Simscape Bus1/LConn3 -- Spatial Contact Force3/RConn1 -- Spatial Contact Force16/RConn1 -- Spatial Contact Force14/RConn1 -- Spatial Contact Force5/RConn1
  Simscape Bus1/LConn4 -- Spatial Contact Force2/RConn1 -- Spatial Contact Force12/RConn1 -- Spatial Contact Force19/RConn1 -- Spatial Contact Force10/RConn1
  Simscape Bus1/LConn5 -- Spatial Contact Force15/RConn1 -- Spatial Contact Force17/RConn1 -- Spatial Contact Force8/RConn1 -- Spatial Contact Force6/RConn1

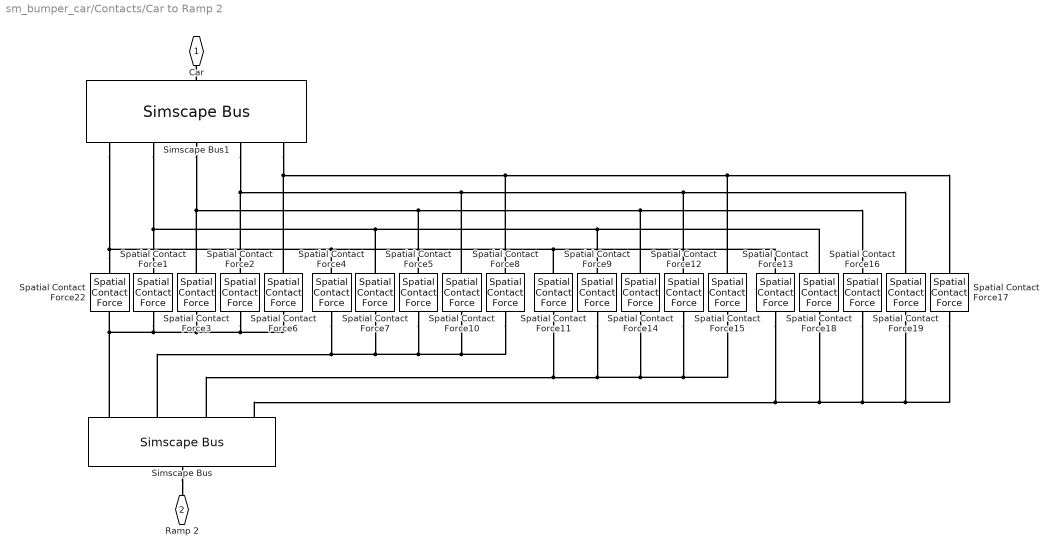
== system sm_bumper_car/Contacts/Car to Ramp 2 ==
  Simscape Bus : SimscapeBus  HierarchyStrings=Incline;BackStop;LeftRail;RightRail
  Simscape Bus1 : SimscapeBus  HierarchyStrings=Body;BackLeft;BackRight;FrontLeft;FrontRight
  Spatial Contact Force{1..19,22} (20 alike) : sm_lib/Forces and Torques/Spatial Contact Force  CoefficientOfDynamicFriction=muk  CoefficientOfStaticFriction=mus  SenseContactBaseRotation=off  SenseContactBaseTranslation=off  NormalDamping=b  NormalDampingUnits=N/(m/s)  SenseContactFollowerRotation=off  SenseContactFollowerTranslation=off  SenseContactSignal=off  NormalStiffness=k  NormalStiffnessUnits=N/m  FrictionalCriticalVelocity=cv  FrictionalCriticalVelocityUnits=m/s  ZeroCrossDetectContactStartAndEnd=off  FrictionType=SmoothStickSlip  SenseFrictionalForceMagnitude=off  SenseNormalForceMagnitude=off  NormalForceType=SmoothSpringDamper  SenseNormalVelocity=off  SenseSeparationDistance=off  SenseTangentialVelocity=off  SenseTangentialVelocityMagnitude=off  NormalTransitionRegionWidth=tau  NormalTransitionRegionWidthUnits=m
  Car : PMIOPort  Side=Right
  Ramp 2 : PMIOPort  Port=2  Side=Left
  connections:
  Spatial Contact Force3/LConn1 -- Spatial Contact Force1/LConn1 -- Spatial Contact Force22/LConn1 -- Simscape Bus/LConn1 -- Spatial Contact Force6/LConn1 -- Spatial Contact Force2/LConn1
  Simscape Bus/LConn2 -- Spatial Contact Force4/LConn1 -- Spatial Contact Force7/LConn1 -- Spatial Contact Force5/LConn1 -- Spatial Contact Force8/LConn1 -- Spatial Contact Force10/LConn1
  Spatial Contact Force14/LConn1 -- Spatial Contact Force12/LConn1 -- Spatial Contact Force15/LConn1 -- Spatial Contact Force9/LConn1 -- Simscape Bus/LConn3 -- Spatial Contact Force11/LConn1
  Simscape Bus/LConn4 -- Spatial Contact Force13/LConn1 -- Spatial Contact Force16/LConn1 -- Spatial Contact Force19/LConn1 -- Spatial Contact Force17/LConn1 -- Spatial Contact Force18/LConn1
  Simscape Bus/RConn1 -- Ramp 2/RConn1
  Simscape Bus1/RConn1 -- Car/RConn1
  Spatial Contact Force22/RConn1 -- Simscape Bus1/LConn1 -- Spatial Contact Force4/RConn1 -- Spatial Contact Force13/RConn1 -- Spatial Contact Force11/RConn1
  Spatial Contact Force1/RConn1 -- Simscape Bus1/LConn2 -- Spatial Contact Force7/RConn1 -- Spatial Contact Force9/RConn1 -- Spatial Contact Force18/RConn1
  Simscape Bus1/LConn3 -- Spatial Contact Force16/RConn1 -- Spatial Contact Force14/RConn1 -- Spatial Contact Force5/RConn1 -- Spatial Contact Force3/RConn1
  Spatial Contact Force12/RConn1 -- Spatial Contact Force19/RConn1 -- Spatial Contact Force10/RConn1 -- Simscape Bus1/LConn4 -- Spatial Contact Force2/RConn1
  Spatial Contact Force15/RConn1 -- Spatial Contact Force17/RConn1 -- Spatial Contact Force8/RConn1 -- Spatial Contact Force6/RConn1 -- Simscape Bus1/LConn5

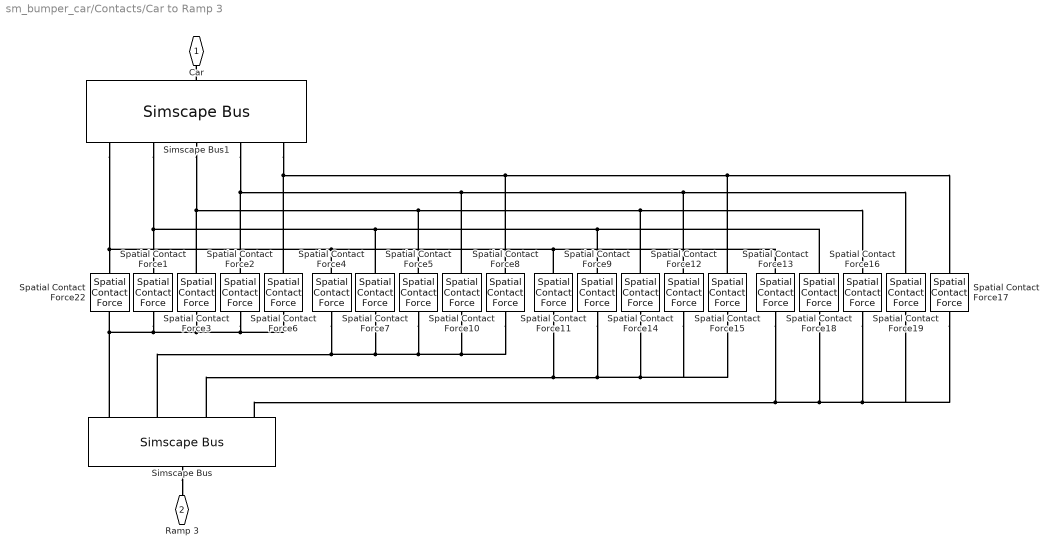
== system sm_bumper_car/Contacts/Car to Ramp 3 ==
  Simscape Bus : SimscapeBus  HierarchyStrings=Incline;BackStop;LeftRail;RightRail
  Simscape Bus1 : SimscapeBus  HierarchyStrings=Body;BackLeft;BackRight;FrontLeft;FrontRight
  Spatial Contact Force{1..19,22} (20 alike) : sm_lib/Forces and Torques/Spatial Contact Force  CoefficientOfDynamicFriction=muk  CoefficientOfStaticFriction=mus  SenseContactBaseRotation=off  SenseContactBaseTranslation=off  NormalDamping=b  NormalDampingUnits=N/(m/s)  SenseContactFollowerRotation=off  SenseContactFollowerTranslation=off  SenseContactSignal=off  NormalStiffness=k  NormalStiffnessUnits=N/m  FrictionalCriticalVelocity=cv  FrictionalCriticalVelocityUnits=m/s  ZeroCrossDetectContactStartAndEnd=off  FrictionType=SmoothStickSlip  SenseFrictionalForceMagnitude=off  SenseNormalForceMagnitude=off  NormalForceType=SmoothSpringDamper  SenseNormalVelocity=off  SenseSeparationDistance=off  SenseTangentialVelocity=off  SenseTangentialVelocityMagnitude=off  NormalTransitionRegionWidth=tau  NormalTransitionRegionWidthUnits=m
  Car : PMIOPort  Side=Right
  Ramp 3 : PMIOPort  Port=2  Side=Left
  connections:
  Simscape Bus1/LConn5 -- Spatial Contact Force6/RConn1 -- Spatial Contact Force8/RConn1 -- Spatial Contact Force17/RConn1 -- Spatial Contact Force15/RConn1
  Spatial Contact Force2/RConn1 -- Simscape Bus1/LConn4 -- Spatial Contact Force10/RConn1 -- Spatial Contact Force19/RConn1 -- Spatial Contact Force12/RConn1
  Spatial Contact Force3/RConn1 -- Spatial Contact Force5/RConn1 -- Spatial Contact Force14/RConn1 -- Spatial Contact Force16/RConn1 -- Simscape Bus1/LConn3
  Spatial Contact Force18/RConn1 -- Spatial Contact Force9/RConn1 -- Spatial Contact Force7/RConn1 -- Simscape Bus1/LConn2 -- Spatial Contact Force1/RConn1
  Spatial Contact Force11/RConn1 -- Spatial Contact Force13/RConn1 -- Spatial Contact Force4/RConn1 -- Simscape Bus1/LConn1 -- Spatial Contact Force22/RConn1
  Simscape Bus1/RConn1 -- Car/RConn1
  Simscape Bus/RConn1 -- Ramp 3/RConn1
  Spatial Contact Force18/LConn1 -- Spatial Contact Force17/LConn1 -- Spatial Contact Force19/LConn1 -- Spatial Contact Force16/LConn1 -- Spatial Contact Force13/LConn1 -- Simscape Bus/LConn4
  Spatial Contact Force11/LConn1 -- Simscape Bus/LConn3 -- Spatial Contact Force9/LConn1 -- Spatial Contact Force15/LConn1 -- Spatial Contact Force12/LConn1 -- Spatial Contact Force14/LConn1
  Spatial Contact Force10/LConn1 -- Spatial Contact Force8/LConn1 -- Spatial Contact Force5/LConn1 -- Spatial Contact Force7/LConn1 -- Spatial Contact Force4/LConn1 -- Simscape Bus/LConn2
  Spatial Contact Force2/LConn1 -- Spatial Contact Force6/LConn1 -- Simscape Bus/LConn1 -- Spatial Contact Force22/LConn1 -- Spatial Contact Force1/LConn1 -- Spatial Contact Force3/LConn1

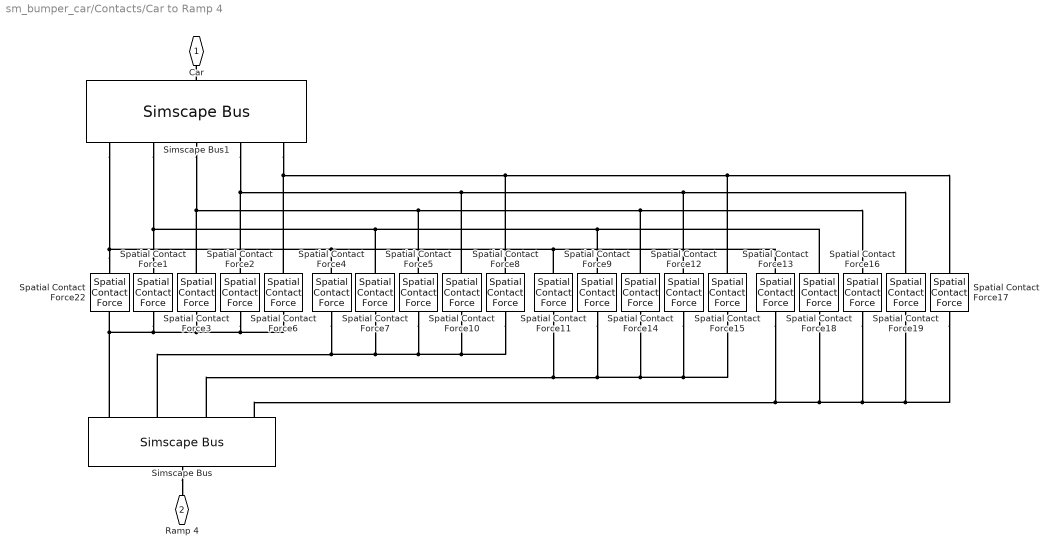
== system sm_bumper_car/Contacts/Car to Ramp 4 ==
  Simscape Bus : SimscapeBus  HierarchyStrings=Incline;BackStop;LeftRail;RightRail
  Simscape Bus1 : SimscapeBus  HierarchyStrings=Body;BackLeft;BackRight;FrontLeft;FrontRight
  Spatial Contact Force{1..19,22} (20 alike) : sm_lib/Forces and Torques/Spatial Contact Force  CoefficientOfDynamicFriction=muk  CoefficientOfStaticFriction=mus  SenseContactBaseRotation=off  SenseContactBaseTranslation=off  NormalDamping=b  NormalDampingUnits=N/(m/s)  SenseContactFollowerRotation=off  SenseContactFollowerTranslation=off  SenseContactSignal=off  NormalStiffness=k  NormalStiffnessUnits=N/m  FrictionalCriticalVelocity=cv  FrictionalCriticalVelocityUnits=m/s  ZeroCrossDetectContactStartAndEnd=off  FrictionType=SmoothStickSlip  SenseFrictionalForceMagnitude=off  SenseNormalForceMagnitude=off  NormalForceType=SmoothSpringDamper  SenseNormalVelocity=off  SenseSeparationDistance=off  SenseTangentialVelocity=off  SenseTangentialVelocityMagnitude=off  NormalTransitionRegionWidth=tau  NormalTransitionRegionWidthUnits=m
  Car : PMIOPort  Side=Right
  Ramp 4 : PMIOPort  Port=2  Side=Left
  connections:
  Spatial Contact Force3/LConn1 -- Spatial Contact Force1/LConn1 -- Spatial Contact Force22/LConn1 -- Simscape Bus/LConn1 -- Spatial Contact Force6/LConn1 -- Spatial Contact Force2/LConn1
  Simscape Bus/LConn2 -- Spatial Contact Force4/LConn1 -- Spatial Contact Force7/LConn1 -- Spatial Contact Force5/LConn1 -- Spatial Contact Force8/LConn1 -- Spatial Contact Force10/LConn1
  Spatial Contact Force14/LConn1 -- Spatial Contact Force12/LConn1 -- Spatial Contact Force15/LConn1 -- Spatial Contact Force9/LConn1 -- Simscape Bus/LConn3 -- Spatial Contact Force11/LConn1
  Simscape Bus/LConn4 -- Spatial Contact Force13/LConn1 -- Spatial Contact Force16/LConn1 -- Spatial Contact Force19/LConn1 -- Spatial Contact Force17/LConn1 -- Spatial Contact Force18/LConn1
  Simscape Bus/RConn1 -- Ramp 4/RConn1
  Simscape Bus1/RConn1 -- Car/RConn1
  Spatial Contact Force22/RConn1 -- Simscape Bus1/LConn1 -- Spatial Contact Force4/RConn1 -- Spatial Contact Force13/RConn1 -- Spatial Contact Force11/RConn1
  Spatial Contact Force1/RConn1 -- Simscape Bus1/LConn2 -- Spatial Contact Force7/RConn1 -- Spatial Contact Force9/RConn1 -- Spatial Contact Force18/RConn1
  Simscape Bus1/LConn3 -- Spatial Contact Force16/RConn1 -- Spatial Contact Force14/RConn1 -- Spatial Contact Force5/RConn1 -- Spatial Contact Force3/RConn1
  Spatial Contact Force12/RConn1 -- Spatial Contact Force19/RConn1 -- Spatial Contact Force10/RConn1 -- Simscape Bus1/LConn4 -- Spatial Contact Force2/RConn1
  Spatial Contact Force15/RConn1 -- Spatial Contact Force17/RConn1 -- Spatial Contact Force8/RConn1 -- Spatial Contact Force6/RConn1 -- Simscape Bus1/LConn5
